simulink model "Project_Mobius"  (R2023b)
settings: Solver=ode4  StartTime=0.0  StopTime=100  FixedStep=5e-3  RelTol=1e-3
values from neighbouring files (symbols this model uses):
  aileron_stuck = 0.1    [fault_insertion.m]
  aircraft_b = 2    [initial.m]
  aircraft_c = 0.275    [initial.m]
  aircraft_mass = 6.031    [initial.m]
  c1 = ((Iyy - Izz)*Izz - Ixz*Ixz)/sigma    (= -0.404494382022)    [initial.m]
  c2 = ((Ixx - Iyy + Izz)*Ixz)/sigma    (= 0)    [initial.m]
  c3 = Izz/sigma    (= 3.74531835206)    [initial.m]
  c4 = Ixz/sigma    (= 0)    [initial.m]
  c5 = (Izz - Ixx)/Iyy    (= 0.404494382022)    [initial.m]
  c6 = Ixz/Iyy    (= 0)    [initial.m]
  c7 = 1/Iyy    (= 3.74531835206)    [initial.m]
  c8 = (Ixx*(Ixx - Iyy) + Ixz*Ixz)/sigma    (= 0)    [initial.m]
  c9 = Ixx/sigma    (= 2.66666666667)    [initial.m]
  CD_fuselage = 0.027    [initial.m]
  CdDa = 0.092132    [initial.m]
  CdDe = 0.016043    [initial.m]
  CdDr = 0.0097403    [initial.m]
  CDmin = 0.06047    [initial.m]
  CL0 = 0.81857    [initial.m]
  CL_CDmin = 0.4806    [initial.m]
  CLa = 4.09127    [initial.m]
  CLa_dot = 0    [initial.m]
  Clb = -0.00161    [initial.m]
  ClDa = 0.286593    [initial.m]
  CLDa = -0.85291    [initial.m]
  CLDe = 0.50787    [initial.m]
  ClDr = 0.013407    [initial.m]
  Clp = -0.47584    [initial.m]
  CLq = 7.31097    [initial.m]
  Clr = 0.27153    [initial.m]
  Cm0 = 0.00763    [initial.m]
  Cma = -1.76966    [initial.m]
  CmDe = -1.83747    [initial.m]
  Cmq = -19.22663    [initial.m]
  Cnb = 0.0918    [initial.m]
  CnDa = 0.0049274    [initial.m]
  CnDr = -0.067036    [initial.m]
  Cnp = -0.13267    [initial.m]
  Cnr = -0.08829    [initial.m]
  CYb = -0.00157    [initial.m]
  CYDr = 0.128915    [initial.m]
  CYp = -0.00157    [initial.m]
  CYr = 0.18368    [initial.m]
  elevator_stuck = 0    [fault_insertion.m]
  fault_time_start = 1    [fault_insertion.m]
  flight_mode = 1    [initial.m]
  g = 9.8060    (= 9.806)    [initial.m]
  init_alpha = alpha_trim    (= 0)    [initial.m]
  init_h = 10    [initial.m]
  init_p = 0    [initial.m]
  init_phi = 0    [initial.m]
  init_psi = 0    [initial.m]
  init_q = 0    [initial.m]
  init_r = 0    [initial.m]
  init_theta = init_alpha    (= 0)    [initial.m]
  init_u = Vb(1)    [initial.m]
  init_v = Vb(2)    [initial.m]
  init_w = Vb(3)    [initial.m]
  init_x = 0    [initial.m]
  init_y = 0    [initial.m]
  K = 0.1328    [initial.m]
  Max_RPM = 10000    [initial.m]
  p_sensor_fault = 0    [fault_insertion.m]
  phi_sensor_fault = 0    [fault_insertion.m]
  PropDiameter = 0.3052    [initial.m]
  psi_sensor_fault = 0    [fault_insertion.m]
  q_sensor_fault = 0    [fault_insertion.m]
  r_sensor_fault = 0    [fault_insertion.m]
  rho = 1.2250    (= 1.225)    [initial.m]
  rotor1_direction = 1    [initial.m]
  rotor1_fail = 0    [fault_insertion.m]
  rotor2_direction = -1    [initial.m]
  rotor2_fail = 0    [fault_insertion.m]
  rotor3_direction = -1    [initial.m]
  rotor3_fail = 0    [fault_insertion.m]
  rotor4_direction = 1    [initial.m]
  rotor4_fail = 0    [fault_insertion.m]
  rotor_arm1 = [0.375,0.375,0]    [initial.m]
  rotor_arm2 = [0.375,-0.375,0]    [initial.m]
  rotor_arm3 = [-0.375,-0.375,0]    [initial.m]
  rotor_arm4 = [-0.375,0.375,0]    [initial.m]
  RPM1_init = rotor_n * 60    (= 5940)    [initial.m]
  RPM2_init = rotor_n * 60    (= 5940)    [initial.m]
  RPM3_init = 0    [initial.m]
  RPM4_init = 0    [initial.m]
  rudder_stuck = 0    [fault_insertion.m]
  theta_sensor_fault = 0    [fault_insertion.m]
  tilt1_fail = 0    [fault_insertion.m]
  tilt1_init = lambda    [initial.m]
  tilt2_fail = 0    [fault_insertion.m]
  tilt2_init = lambda    [initial.m]
  tilt3_init = 0    [initial.m]
  tilt4_init = 0    [initial.m]
  u_sensor_fault = 0    [fault_insertion.m]
  v_sensor_fault = 0    [fault_insertion.m]
  w_sensor_fault = 0    [fault_insertion.m]
undefined symbols (not defined in the file or in its folder): FixedWingMission, HoverMission
libraries: slpidlib x20, simulink_extras x12, simulink x7, aerolibasang x6, matrix_library x4, uavalgslib x4, sharedutil x1, sharedtransform x1
(part 3 of 4)

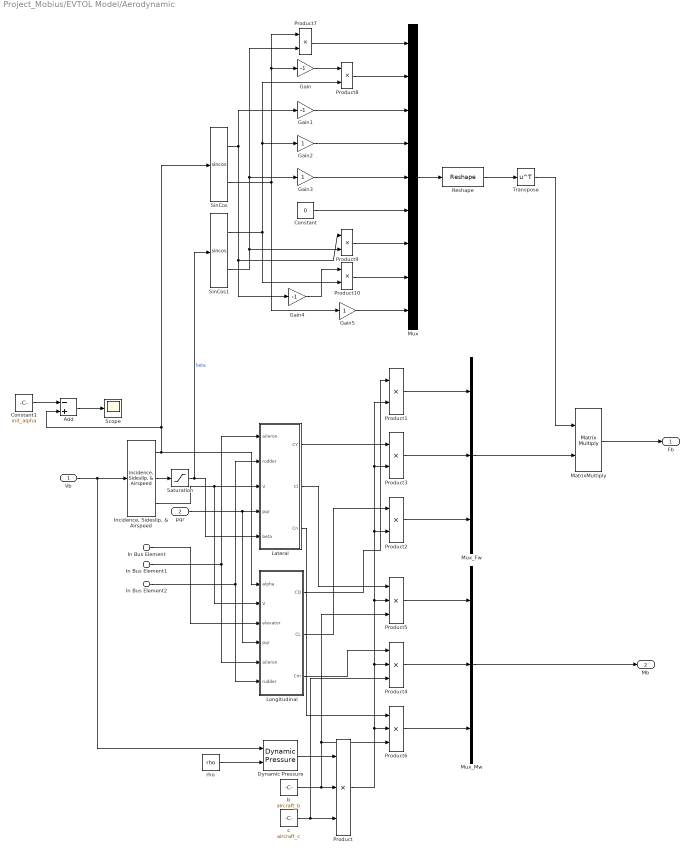
== system Project_Mobius/EVTOL Model/Aerodynamic ==
  Vb : Inport
  pqr : Inport  Port=2
  In Bus Element : Inport  Port=3  PortName=CtrlSurfaces  Element=Elevator
  In Bus Element1 : Inport  Port=3  PortName=CtrlSurfaces  Element=Aileron
  In Bus Element2 : Inport  Port=3  PortName=CtrlSurfaces  Element=Rudder
  Add : Sum  Inputs=-+
  Constant : Constant  Value=0
  Constant1 : Constant  Value=init_alpha
  Dynamic Pressure : aerolibasang/Dynamic Pressure
  Gain : Gain  Gain=-1
  Gain1 : Gain  Gain=-1
  Gain2 : Gain
  Gain3 : Gain
  Gain4 : Gain  Gain=-1
  Gain5 : Gain
  "Incidence, Sideslip, & Airspeed" : aerolibasang/Incidence, Sideslip, & Airspeed
  Lateral : Subsystem
  Longitudinal : Subsystem
  MatrixMultiply : Product  Multiplication=Matrix(*)
  Mux : Mux  Inputs=9
  Mux_Fw : Mux  Inputs=3
  Mux_Mw : Mux  Inputs=3
  Product{,4..6} (4 alike) : Product  Inputs=3
  Product{1..3,7..10} (7 alike) : Product
  Reshape : Reshape  OutputDimensionality=Customize  OutputDimensions=[3,3]
  Saturation : Saturate  UpperLimit=14*pi/180  LowerLimit=-14*pi/180
  Scope : Scope
  SinCos : Trigonometry  Operator=sincos
  SinCos1 : Trigonometry  Operator=sincos
  Transpose : Math  Operator=transpose
  b : Constant  Value=aircraft_b
  c : Constant  Value=aircraft_c
  rho : Constant  Value=rho
  Fb : Outport
  Mb : Outport  Port=2
  wires:
  Vb/1 -> "Incidence, Sideslip, & Airspeed"/1, Dynamic Pressure/1
  rho/1 -> Dynamic Pressure/2
  In Bus Element1/1 -> Longitudinal/5(aileron), Lateral/1(aileron)
  In Bus Element2/1 -> Longitudinal/6(rudder), Lateral/2(rudder)
  "Incidence, Sideslip, & Airspeed"/3 -> Longitudinal/2(V), Lateral/3(V)
  pqr/1 -> Longitudinal/4(pqr), Lateral/4(pqr)
  "Incidence, Sideslip, & Airspeed"/2 -> Saturation/1
  "Incidence, Sideslip, & Airspeed"/1 -> Add/2, SinCos/1, Longitudinal/1(alpha)
  In Bus Element/1 -> Longitudinal/3(elevator)
  Dynamic Pressure/1 -> Product/1
  b/1 -> Product6/3, Product5/3, Product/2
  c/1 -> Product4/3, Product/3
  Longitudinal/1(CD) -> Product1/1
  Product/1 -> Product2/2, Product3/2, Product1/2, Product5/2, Product4/2, Product6/2
  Longitudinal/2(CL) -> Product2/1
  Lateral/1(CY) -> Product3/1
  Longitudinal/3(Cm) -> Product4/1
  Lateral/2(Cl) -> Product5/1
  Lateral/3(Cn) -> Product6/1
  Product3/1 -> Mux_Fw/2
  Product2/1 -> Mux_Fw/3
  Product1/1 -> Mux_Fw/1
  Mux_Fw/1 -> MatrixMultiply/2
  Product5/1 -> Mux_Mw/1
  Product4/1 -> Mux_Mw/2
  Product6/1 -> Mux_Mw/3
  SinCos/2 -> Gain5/1, Gain/1, Product7/1
  SinCos1/2 -> Product9/2, Gain3/1, Product7/2
  Gain/1 -> Product8/1
  SinCos1/1 -> Product10/2, Gain2/1, Product8/2
  SinCos/1 -> Gain1/1, Product9/1, Gain4/1
  Gain4/1 -> Product10/1
  Product7/1 -> Mux/1
  Product8/1 -> Mux/2
  Gain1/1 -> Mux/3
  Gain2/1 -> Mux/4
  Gain3/1 -> Mux/5
  Constant/1 -> Mux/6
  Product9/1 -> Mux/7
  Product10/1 -> Mux/8
  Gain5/1 -> Mux/9
  Mux/1 -> Reshape/1
  MatrixMultiply/1 -> Fb/1
  Reshape/1 -> Transpose/1
  Transpose/1 -> MatrixMultiply/1
  Mux_Mw/1 -> Mb/1
  Saturation/1 -> SinCos1/1, Lateral/5(beta)  "beta"
  Constant1/1 -> Add/1
  Add/1 -> Scope/1

== system Project_Mobius/EVTOL Model/Fuselage Drag ==
  Vb : Inport
  Add : Sum  Inputs=+++
  Constant : Constant  Value=CD_fuselage
  Demux : Demux  Outputs=3
  Gain : Gain  Gain=-1
  Product : Product
  Product1 : Product
  Sqrt : Sqrt
  Square : Math  Operator=square
  Square1 : Math  Operator=square
  Square2 : Math  Operator=square
  FD,fuselage : Outport
  wires:
  Vb/1 -> Product1/2, Demux/1
  Demux/1 -> Square/1
  Demux/2 -> Square1/1
  Demux/3 -> Square2/1
  Square/1 -> Add/1
  Square1/1 -> Add/2
  Square2/1 -> Add/3
  Add/1 -> Sqrt/1
  Sqrt/1 -> Product/2
  Constant/1 -> Product/1
  Product/1 -> Product1/1
  Product1/1 -> Gain/1
  Gain/1 -> FD,fuselage/1

== system Project_Mobius/EVTOL Model/Gravity ==
  Attitude : Inport
  Demux : Demux  Outputs=3
  Gain : Gain  Gain=-1
  Gain1 : Gain  Gain=aircraft_mass*g
  Mux : Mux  Inputs=3
  Product : Product
  Product1 : Product
  SinCos : Trigonometry  Operator=sincos
  SinCos1 : Trigonometry  Operator=sincos
  Fb : Outport
  wires:
  Attitude/1 -> Demux/1
  Demux/1 -> SinCos/1
  Demux/2 -> SinCos1/1
  SinCos1/2 -> Product/2, Product1/1
  SinCos/1 -> Product/1
  SinCos/2 -> Product1/2
  SinCos1/1 -> Gain/1
  Gain/1 -> Mux/1
  Product/1 -> Mux/2
  Product1/1 -> Mux/3
  Mux/1 -> Gain1/1
  Gain1/1 -> Fb/1

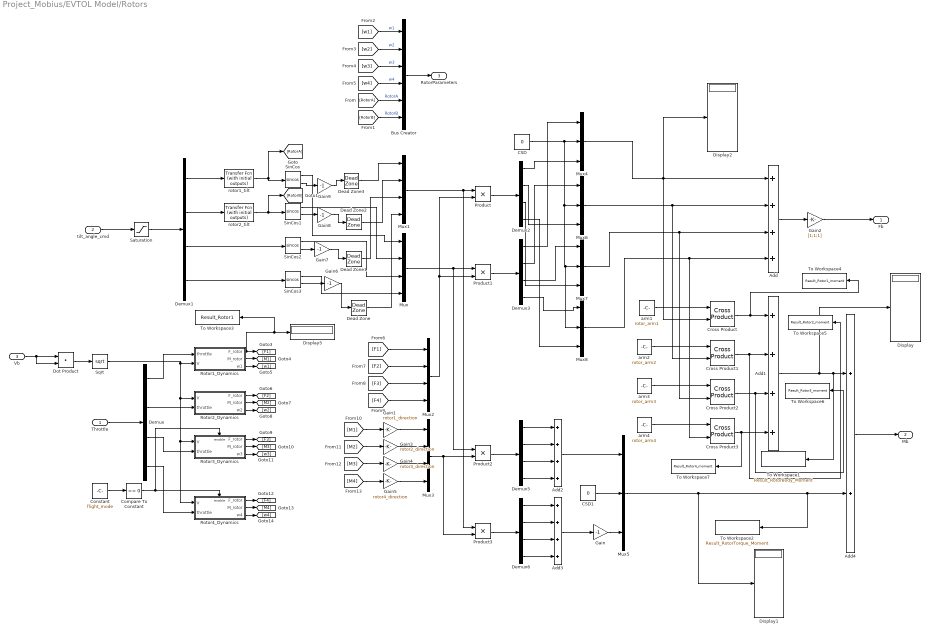
== system Project_Mobius/EVTOL Model/Rotors ==
  Throttle : Inport
  tilt_angle_cmd : Inport  Port=2
  Vb : Inport  Port=3
  Add{,1..3} (4 alike) : Sum  Inputs=++++
  Add4 : Sum
  Bus Creator : BusCreator  Inputs=6
  CSD : Constant  Value=0
  CSD1 : Constant  Value=0
  Compare To Constant : simulink/Logic and Bit Operations/Compare To Constant  relop===  const=0  OutDataTypeStr=boolean
  Constant : Constant  Value=flight_mode
  Cross Product{,1..3} (4 alike) : matrix_library/Cross Product
  Dead Zone{,1..3} (4 alike) : DeadZone  LowerValue=-cos(pi/2)  UpperValue=cos(pi/2)
  Demux{,1..3,5..6} (6 alike) : Demux
  Display{,1..2,5} (4 alike) : Display
  Dot Product : DotProduct  OutDataTypeStr=Inherit: Inherit via internal rule
  Gain{,6..9} (5 alike) : Gain  Gain=-1
  Gain1 : Gain  Gain=rotor1_direction
  Gain2 : Gain  Gain=[1;1;1]
  Gain3 : Gain  Gain=rotor2_direction
  Gain4 : Gain  Gain=rotor3_direction
  Gain5 : Gain  Gain=rotor4_direction
  Mux{,1..3} (4 alike) : Mux
  Mux{4..8} (5 alike) : Mux  Inputs=3
  Product{,1..3} (4 alike) : Product
  Rotor1_Dynamics : Subsystem
  Rotor2_Dynamics : Subsystem
  Rotor3_Dynamics : Subsystem
  Rotor4_Dynamics : Subsystem
  Saturation : Saturate  UpperLimit=90*pi/180  LowerLimit=-90*pi/180
  SinCos{,1..3} (4 alike) : Trigonometry  Operator=sincos
  Sqrt : Sqrt
  To Workspace1 : ToWorkspace  VariableName=Result_RotorBody_Moment  SampleTime=0.005
  To Workspace2 : ToWorkspace  VariableName=Result_RotorTorque_Moment  SampleTime=0.005
  To Workspace3 : ToWorkspace  VariableName=Result_Rotor1  SampleTime=0.005
  To Workspace4 : ToWorkspace  VariableName=Result_Rotor1_moment  SampleTime=0.005
  To Workspace5 : ToWorkspace  VariableName=Result_Rotor2_moment  SampleTime=0.005
  To Workspace6 : ToWorkspace  VariableName=Result_Rotor3_moment  SampleTime=0.005
  To Workspace7 : ToWorkspace  VariableName=Result_Rotor4_moment  SampleTime=0.005
  arm1 : Constant  Value=rotor_arm1
  arm2 : Constant  Value=rotor_arm2
  arm3 : Constant  Value=rotor_arm3
  arm4 : Constant  Value=rotor_arm4
  rotor1_tilt : simulink_extras/Additional Linear/Transfer Fcn (with initial outputs)  N=[1]  D="[0.1  1]"  Y0=tilt1_init  U0=tilt1_init
  rotor2_tilt : simulink_extras/Additional Linear/Transfer Fcn (with initial outputs)  N=[1]  D="[0.1  1]"  Y0=tilt2_init  U0=tilt2_init
  Fb : Outport
  Mb : Outport  Port=2
  RotorParameters : Outport  Port=3
  wires:
  Throttle/1 -> Demux/1
  Demux/1 -> Rotor1_Dynamics/1(throttle)
  Demux1/1 -> rotor1_tilt/1
  Demux1/2 -> rotor2_tilt/1
  tilt_angle_cmd/1 -> Saturation/1
  Saturation/1 -> Demux1/1
  rotor1_tilt/1 -> [RotorA], SinCos/1
  rotor2_tilt/1 -> [RotorB], SinCos1/1
  Demux1/3 -> SinCos2/1
  Demux1/4 -> SinCos3/1
  SinCos/1 -> Mux/1
  SinCos1/1 -> Mux/2
  SinCos2/1 -> Mux/3
  SinCos3/1 -> Mux/4
  SinCos1/2 -> Gain8/1
  SinCos3/2 -> Gain6/1
  Mux2/1 -> Product1/2, Product/2
  Product/1 -> Demux2/1
  Product1/1 -> Demux3/1
  Add/1 -> Gain2/1
  Mux3/1 -> Product3/2, Product2/2
  Mux/1 -> Product2/1, Product1/1
  Product2/1 -> Demux5/1
  Product3/1 -> Demux6/1
  Demux5/1 -> Add2/1
  Demux5/2 -> Add2/2
  Demux5/3 -> Add2/3
  Demux5/4 -> Add2/4
  Demux6/1 -> Add3/1
  Demux6/2 -> Add3/2
  Demux6/3 -> Add3/3
  Demux6/4 -> Add3/4
  Add3/1 -> Gain/1
  Add2/1 -> Mux5/1
  CSD1/1 -> Mux5/2
  CSD/1 -> Mux8/2, Mux7/2, Mux6/2, Mux4/2
  Mux7/1 -> Add/3, Cross Product2/2
  Mux8/1 -> Cross Product3/2, Add/4
  arm1/1 -> Cross Product/1
  arm2/1 -> Cross Product1/1
  Mux6/1 -> Add/2, Cross Product1/2
  arm3/1 -> Cross Product2/1
  arm4/1 -> Cross Product3/1
  Cross Product/1 -> To Workspace4/1, Add1/1
  Cross Product1/1 -> To Workspace5/1, Add1/2
  Cross Product2/1 -> To Workspace6/1, Add1/3
  Cross Product3/1 -> Add1/4, To Workspace7/1
  Add1/1 -> Display/1, To Workspace1/1, Add4/1
  Mux5/1 -> Display1/1, To Workspace2/1, Add4/2
  Add4/1 -> Mb/1
  Gain2/1 -> Fb/1
  Vb/1 -> Dot Product/2, Dot Product/1
  Dot Product/1 -> Sqrt/1
  Sqrt/1 -> Rotor4_Dynamics/1(V), Rotor3_Dynamics/1(V), Rotor2_Dynamics/1(V), Rotor1_Dynamics/2(V)
  Demux/2 -> Rotor2_Dynamics/2(throttle)
  Demux/3 -> Rotor3_Dynamics/2(throttle)
  Demux/4 -> Rotor4_Dynamics/2(throttle)
  Demux3/1 -> Mux4/1
  Demux3/2 -> Mux6/1
  Demux3/3 -> Mux7/1
  Demux3/4 -> Mux8/1
  Demux2/1 -> Mux4/3
  Demux2/2 -> Mux6/3
  Demux2/3 -> Mux7/3
  Demux2/4 -> Mux8/3
  Gain/1 -> Mux5/3
  Gain3/1 -> Mux3/2
  Gain4/1 -> Mux3/3
  Gain5/1 -> Mux3/4
  Mux1/1 -> Product3/1, Product/1
  Compare To Constant/1 -> Rotor4_Dynamics/Enable, Rotor3_Dynamics/Enable
  Dead Zone/1 -> Mux1/4
  SinCos2/2 -> Gain7/1
  Dead Zone1/1 -> Mux1/3
  Dead Zone2/1 -> Mux1/2
  Dead Zone3/1 -> Mux1/1
  [w1] -> Bus Creator/1  "w1"
  [w2] -> Bus Creator/2  "w2"
  [w3] -> Bus Creator/3  "w3"
  [w4] -> Bus Creator/4  "w4"
  [RotorA] -> Bus Creator/5  "RotorA"
  [RotorB] -> Bus Creator/6  "RotorB"
  Bus Creator/1 -> RotorParameters/1
  Gain1/1 -> Mux3/1
  Rotor1_Dynamics/1(F_rotor) -> To Workspace3/1, Display5/1, [F1]
  Rotor1_Dynamics/2(M_rotor) -> [M1]
  Rotor1_Dynamics/3(w1) -> [w1]
  Rotor2_Dynamics/1(F_rotor) -> [F2]
  Rotor2_Dynamics/2(M_rotor) -> [M2]
  Rotor2_Dynamics/3(w2) -> [w2]
  Rotor3_Dynamics/1(F_rotor) -> [F3]
  Rotor3_Dynamics/2(M_rotor) -> [M3]
  Rotor3_Dynamics/3(w3) -> [w3]
  Rotor4_Dynamics/1(F_rotor) -> [F4]
  Rotor4_Dynamics/2(M_rotor) -> [M4]
  Rotor4_Dynamics/3(w4) -> [w4]
  [F1] -> Mux2/1
  [F2] -> Mux2/2
  [F3] -> Mux2/3
  [F4] -> Mux2/4
  [M1] -> Gain1/1
  [M2] -> Gain3/1
  [M3] -> Gain4/1
  [M4] -> Gain5/1
  Gain6/1 -> Dead Zone/1
  Gain7/1 -> Dead Zone1/1
  Gain8/1 -> Dead Zone2/1
  SinCos/2 -> Gain9/1
  Gain9/1 -> Dead Zone3/1
  Mux4/1 -> Display2/1, Cross Product/2, Add/1
  Constant/1 -> Compare To Constant/1

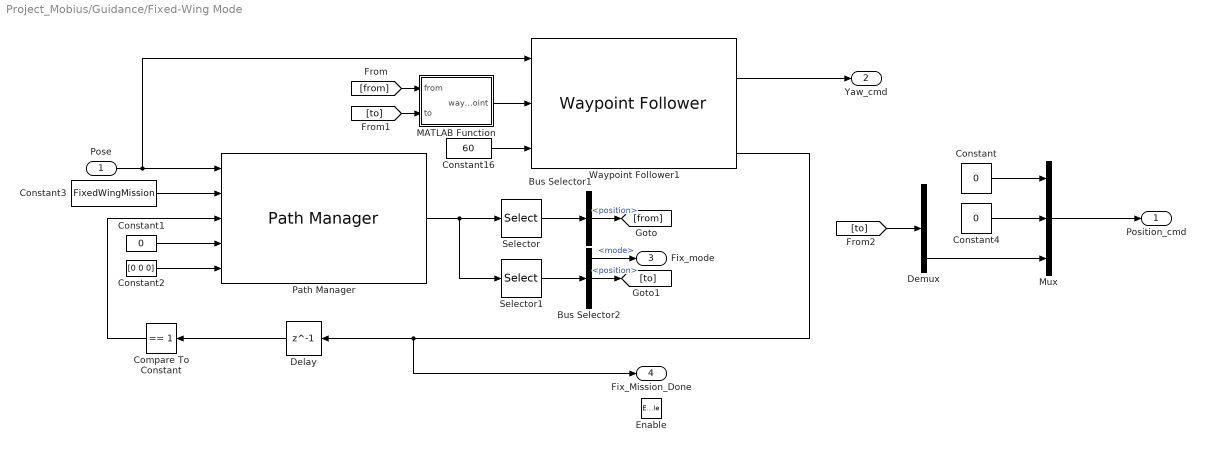
== system Project_Mobius/Guidance/Fixed-Wing Mode ==
  Pose : Inport
  Enable : EnablePort
  Bus Selector1 : BusSelector  OutputSignals=mode,position,params
  Bus Selector2 : BusSelector  OutputSignals=mode,position,params
  Compare To Constant : simulink/Logic and Bit Operations/Compare To Constant  relop===  const=1  OutDataTypeStr=boolean
  Constant : Constant  Value=0
  Constant1 : Constant  Value=0  OutDataTypeStr=uint8
  Constant16 : Constant  Value=60
  Constant2 : Constant  Value=[0 0 0]
  Constant3 : Constant  Value=FixedWingMission  OutDataTypeStr=Bus: doubleUAVPathManagerBus
  Constant4 : Constant  Value=0
  Delay : Delay  DelayLength=1  InitialCondition=0
  Demux : Demux  Outputs=3
  MATLAB Function : MATLAB Function  TreatAsAtomicUnit=on
  Mux : Mux  Inputs=3
  Path Manager : uavalgslib/Path Manager  UAVType=multirotor  LoiterRadius=25  dataType=double  inputBusName='doubleUAVPathManagerBus'  SimulateUsing=Interpreted execution
  Selector : Selector  InputPortWidth=2  IndexOptions=Index vector (dialog)  Indices=2  OutputSizes=1
  Selector1 : Selector  InputPortWidth=2  IndexOptions=Index vector (dialog)  Indices=1  OutputSizes=1
  Waypoint Follower1 : uavalgslib/Waypoint Follower  UAVType=fixed-wing  StartFrom=first  TransitionRadiusSource=internal  TransitionRadius=10  MinLookaheadDistance=60  YawInput=off  ShowCrossTrackErrorOutput=off  ShowStatusOutput=on  SimulateUsing=Code generation
  Position_cmd : Outport
  Yaw_cmd : Outport  Port=2
  Fix_mode : Outport  Port=3
  Fix_Mission_Done : Outport  Port=4
  wires:
  Pose/1 -> Waypoint Follower1/1, Path Manager/1
  MATLAB Function/1(waypoint) -> Waypoint Follower1/2
  Bus Selector1/2 -> [from]  "<position>"
  Waypoint Follower1/5 -> Fix_Mission_Done/1, Delay/1
  Delay/1 -> Compare To Constant/1
  Selector/1 -> Bus Selector1/1
  [from] -> MATLAB Function/1(from)
  Bus Selector2/2 -> [to]  "<position>"
  Constant1/1 -> Path Manager/4
  Constant3/1 -> Path Manager/2
  Constant16/1 -> Waypoint Follower1/3
  Path Manager/1 -> Selector1/1, Selector/1
  [to] -> MATLAB Function/2(to)
  Constant2/1 -> Path Manager/5
  Selector1/1 -> Bus Selector2/1
  Waypoint Follower1/2 -> Yaw_cmd/1
  Mux/1 -> Position_cmd/1
  Constant/1 -> Mux/1
  Constant4/1 -> Mux/2
  [to] -> Demux/1
  Demux/3 -> Mux/3
  Bus Selector2/1 -> Fix_mode/1  "<mode>"
  Compare To Constant/1 -> Path Manager/3

== system Project_Mobius/Guidance/Guidance Command ==
  Desired Position : Inport
  Desired_Course : Inport  Port=2
  Attitude Stablizer : Subsystem
  Bus Creator : BusCreator  Inputs=3
  Constant : Constant  Value=21
  Path_selector : Subsystem
  Command : Outport
  wires:
  Bus Creator/1 -> Command/1
  Attitude Stablizer/1(Attitude) -> [Attitude]  "Attitude"
  Path_selector/1(Xe_cmd) -> [Xe]  "Xe"
  [Attitude] -> Bus Creator/1  "Attitude"
  [Xe] -> Bus Creator/2  "Xe"
  Constant/1 -> Bus Creator/3  "Speed"
  Desired_Course/1 -> Path_selector/1(courseSP)
  Desired Position/1 -> Path_selector/2(positionSP)

== system Project_Mobius/Guidance/MultiRotor Mode ==
  Pose : Inport
  Enable : EnablePort
  Bus Selector1 : BusSelector  OutputSignals=mode,position,params
  Bus Selector2 : BusSelector  OutputSignals=mode,position,params
  Compare To Constant : simulink/Logic and Bit Operations/Compare To Constant  relop===  const=1  OutDataTypeStr=boolean
  Constant : Constant  Value=5
  Constant1 : Constant  Value=0  OutDataTypeStr=uint8
  Constant16 : Constant  Value=5
  Constant2 : Constant  Value=[0 0 0]
  Constant3 : Constant  Value=HoverMission  OutDataTypeStr=Bus: doubleUAVPathManagerBus
  Data Type Conversion : DataTypeConversion  OutDataTypeStr=uint8  SaturateOnIntegerOverflow=off  RndMeth=Floor
  Delay : Delay  DelayLength=1  InitialCondition=0
  Dist2WP : Subsystem
  MATLAB Function : MATLAB Function  TreatAsAtomicUnit=on
  Path Manager : uavalgslib/Path Manager  UAVType=multirotor  LoiterRadius=25  dataType=double  inputBusName='doubleUAVPathManagerBus'  SimulateUsing=Interpreted execution
  Relational Operator1 : RelationalOperator  OutDataTypeStr=boolean  RndMeth=Simplest  InputSameDT=off
  Selector : Selector  InputPortWidth=2  IndexOptions=Index vector (dialog)  Indices=2  OutputSizes=1
  Selector1 : Selector  InputPortWidth=2  IndexOptions=Index vector (dialog)  Indices=1  OutputSizes=1
  Waypoint Follower1 : uavalgslib/Waypoint Follower  UAVType=multirotor  StartFrom=closest  TransitionRadiusSource=internal  TransitionRadius=1  MinLookaheadDistance=0.1  YawInput=on  ShowCrossTrackErrorOutput=off  ShowStatusOutput=off  SimulateUsing=Code generation
  Position_cmd : Outport
  Yaw_cmd : Outport  Port=2
  Hover_mode : Outport  Port=3
  Hover_Mission_Done : Outport  Port=4
  wires:
  Pose/1 -> Dist2WP/3(Pose), Waypoint Follower1/1, Path Manager/1
  MATLAB Function/1(waypoint) -> Waypoint Follower1/2
  Relational Operator1/1 -> Data Type Conversion/1
  Bus Selector1/2 -> [from]  "<position>"
  Data Type Conversion/1 -> Hover_Mission_Done/1, Delay/1
  Compare To Constant/1 -> Path Manager/3
  Selector/1 -> Dist2WP/1(FromWP), Bus Selector1/1
  [from] -> MATLAB Function/1(from)
  Delay/1 -> Compare To Constant/1
  Bus Selector2/2 -> [to]  "<position>"
  Constant1/1 -> Path Manager/4
  Constant3/1 -> Path Manager/2
  Constant/1 -> Relational Operator1/1
  Dist2WP/1(Dist) -> Relational Operator1/2
  Constant16/1 -> Waypoint Follower1/3
  Path Manager/1 -> Selector1/1, Selector/1
  [to] -> MATLAB Function/2(to)
  Constant2/1 -> Path Manager/5
  Bus Selector2/1 -> Hover_mode/1  "<mode>"
  Selector1/1 -> Bus Selector2/1, Dist2WP/2(ToWP)
  Waypoint Follower1/1 -> Position_cmd/1
  Waypoint Follower1/3 -> Yaw_cmd/1

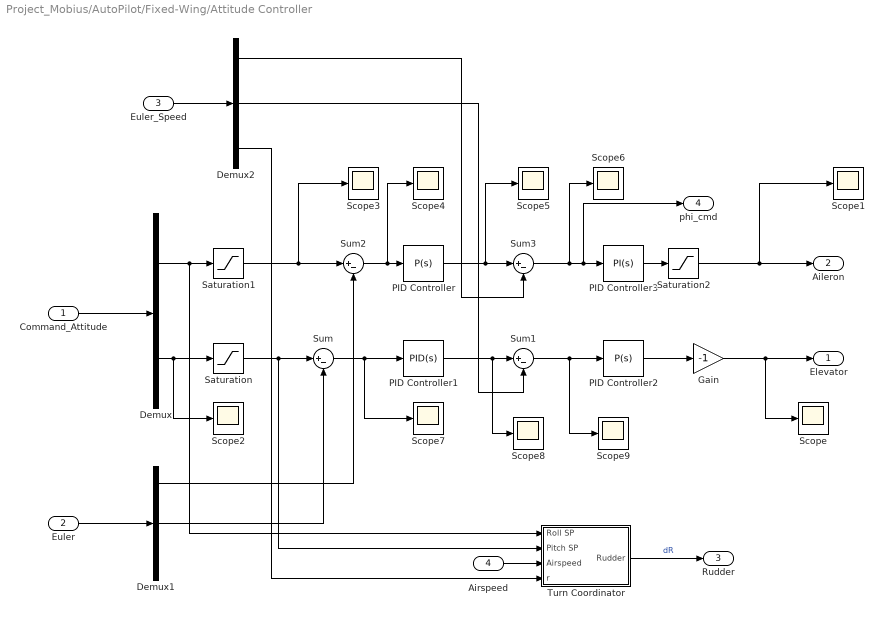
== system Project_Mobius/AutoPilot/Fixed-Wing/Attitude Controller ==
  Command_Attitude : Inport
  Euler : Inport  Port=2
  Euler_Speed : Inport  Port=3
  Airspeed : Inport  Port=4
  Demux : Demux  Outputs=2
  Demux1 : Demux  Outputs=3
  Demux2 : Demux  Outputs=3
  Gain : Gain  Gain=-1
  PID Controller : slpidlib/PID Controller  Controller=P  Form=Parallel  TimeDomain=Continuous-time  UseExternalTs=off  SampleTime=-1  IntegratorMethod=Forward Euler  FilterMethod=Forward Euler  ControllerParametersSource=internal  P=2  I=1  UseKiTs=off  D=0  N=100  UseFilter=on  TunerSelectOption=Transfer Function Based (PID Tuner App)  InitialConditionSource=internal  InitialConditionForIntegrator=0  InitialConditionForFilter=0  DifferentiatorICPrevScaledInput=0  ExternalReset=none  TrackingMode=off  Kt=1  LimitOutput=on  SatLimitsSource=internal  UpperSaturationLimit=1.2277  LowerSaturationLimit=-1.2277  LinearizeAsGain=on  AntiWindupMode=none  Kb=1  LimitIntegrator=off  UpperIntegratorSaturationLimit=inf  LowerIntegratorSaturationLimit=-inf  POutMin=[]  POutMax=[]  IOutMin=[]  IOutMax=[]  DOutMin=[]  DOutMax=[]  NOutMin=[]  NOutMax=[]  SumOutMin=[]  SumOutMax=[]  SaturationOutMin=[]  SaturationOutMax=[]  PParamMin=[]  PParamMax=[]  IParamMin=[]  IParamMax=[]  DParamMin=[]  DParamMax=[]  NParamMin=[]  NParamMax=[]  KbParamMin=[]  KbParamMax=[]  KtParamMin=[]  KtParamMax=[]  KbOutMin=[]  KbOutMax=[]  KtOutMin=[]  KtOutMax=[]  IntegratorOutMin=[]  IntegratorOutMax=[]  FilterOutMin=[]  FilterOutMax=[]  SumI1OutMin=[]  SumI1OutMax=[]  SumI2OutMin=[]  SumI2OutMax=[]  SumI3OutMin=[]  SumI3OutMax=[]  SumI4OutMin=[]  SumI4OutMax=[]  SumDOutMin=[]  SumDOutMax=[]  DifferentiatorOutMin=[]  DifferentiatorOutMax=[]  FilterDiffOutCoefMin=[]  FilterDiffOutCoefMax=[]  ReciprocalOutMin=[]  ReciprocalOutMax=[]  SumDenOutMin=[]  SumDenOutMax=[]  SumNumOutMin=[]  SumNumOutMax=[]  DivideOutMin=[]  DivideOutMax=[]  UdiffTsProdOutMin=[]  UdiffTsProdOutMax=[]  NTsProdOutMin=[]  NTsProdOutMax=[]  UintegralTsProdOutMin=[]  UintegralTsProdOutMax=[]  UngainTsProdOutMin=[]  UngainTsProdOutMax=[]  ClampingZeroOutDataTypeStr=Inherit: Inherit via back propagation  ClampingZeroOutMin=[]  ClampingZeroOutMax=[]  FilterDenConstantOutDataTypeStr=Inherit: Inherit via back propagation  FilterDenConstantOutMin=[]  FilterDenConstantOutMax=[]  PCopyOutDataTypeStr=Inherit: Inherit via back propagation  PCopyOutMin=[]  PCopyOutMax=[]  NCopyOutDataTypeStr=Inherit: Inherit via back propagation  NCopyOutMin=[]  NCopyOutMax=[]  IntegratorContinuousStateAttributes=''  IntegratorStateMustResolveToSignalObject=off  IntegratorRTWStateStorageClass=Auto  FilterContinuousStateAttributes=''  FilterStateMustResolveToSignalObject=off  FilterRTWStateStorageClass=Auto  ParallelPVariant=InternalParameters  IdealPVariant=Disabled  IVariant=Disabled  DVariant=Disabled  IntegratorVariant=Disabled  SatVariant=Enabled  AWVariant=Disabled  PCopyVariant=Disabled  TRVariant=Disabled  FdbkBlocksVariant=Forward  IdealPFdbkVariant=Disabled  SatFdbkVariant=Disabled  DerivativeFilterVariant=Disabled  NVariant=Disabled  NCopyVariant=Disabled_SignalSpec  FilterICVariant=Disabled  IntegratorICVariant=Disabled  ExternalResetVariant=Disabled  TRSumVariant=Passthrough  SumFdbkVariant=Disabled  SumVariant=Passthrough_P  TsampFilterVariant=InternalTs  TsampNgainVariant=Passthrough  TsampIntegralVariant=Disabled_SignalSpec  ExternalSaturationOutDataTypeStr=Inherit: Same as second input
  PID Controller1 : slpidlib/PID Controller  Controller=PID  Form=Parallel  TimeDomain=Continuous-time  UseExternalTs=off  SampleTime=0.05  IntegratorMethod=Forward Euler  FilterMethod=Forward Euler  ControllerParametersSource=internal  P=10  I=0.1  UseKiTs=off  D=0  N=2.2  UseFilter=on  TunerSelectOption=Transfer Function Based (PID Tuner App)  InitialConditionSource=internal  InitialConditionForIntegrator=0  InitialConditionForFilter=0  DifferentiatorICPrevScaledInput=0  ExternalReset=none  TrackingMode=off  Kt=1  LimitOutput=on  SatLimitsSource=internal  UpperSaturationLimit=inf  LowerSaturationLimit=-inf  LinearizeAsGain=on  AntiWindupMode=clamping  Kb=1  LimitIntegrator=off  UpperIntegratorSaturationLimit=inf  LowerIntegratorSaturationLimit=-inf  POutMin=[]  POutMax=[]  IOutMin=[]  IOutMax=[]  DOutMin=[]  DOutMax=[]  NOutMin=[]  NOutMax=[]  SumOutMin=[]  SumOutMax=[]  SaturationOutMin=[]  SaturationOutMax=[]  PParamMin=[]  PParamMax=[]  IParamMin=[]  IParamMax=[]  DParamMin=[]  DParamMax=[]  NParamMin=[]  NParamMax=[]  KbParamMin=[]  KbParamMax=[]  KtParamMin=[]  KtParamMax=[]  KbOutMin=[]  KbOutMax=[]  KtOutMin=[]  KtOutMax=[]  IntegratorOutMin=[]  IntegratorOutMax=[]  FilterOutMin=[]  FilterOutMax=[]  SumI1OutMin=[]  SumI1OutMax=[]  SumI2OutMin=[]  SumI2OutMax=[]  SumI3OutMin=[]  SumI3OutMax=[]  SumI4OutMin=[]  SumI4OutMax=[]  SumDOutMin=[]  SumDOutMax=[]  DifferentiatorOutMin=[]  DifferentiatorOutMax=[]  FilterDiffOutCoefMin=[]  FilterDiffOutCoefMax=[]  ReciprocalOutMin=[]  ReciprocalOutMax=[]  SumDenOutMin=[]  SumDenOutMax=[]  SumNumOutMin=[]  SumNumOutMax=[]  DivideOutMin=[]  DivideOutMax=[]  UdiffTsProdOutMin=[]  UdiffTsProdOutMax=[]  NTsProdOutMin=[]  NTsProdOutMax=[]  UintegralTsProdOutMin=[]  UintegralTsProdOutMax=[]  UngainTsProdOutMin=[]  UngainTsProdOutMax=[]  ClampingZeroOutDataTypeStr=Inherit: Inherit via back propagation  ClampingZeroOutMin=[]  ClampingZeroOutMax=[]  FilterDenConstantOutDataTypeStr=Inherit: Inherit via back propagation  FilterDenConstantOutMin=[]  FilterDenConstantOutMax=[]  PCopyOutDataTypeStr=Inherit: Inherit via back propagation  PCopyOutMin=[]  PCopyOutMax=[]  NCopyOutDataTypeStr=Inherit: Inherit via back propagation  NCopyOutMin=[]  NCopyOutMax=[]  IntegratorContinuousStateAttributes=''  IntegratorStateMustResolveToSignalObject=off  IntegratorRTWStateStorageClass=Auto  FilterContinuousStateAttributes=''  FilterStateMustResolveToSignalObject=off  FilterRTWStateStorageClass=Auto  ParallelPVariant=InternalParameters  IdealPVariant=Disabled  IVariant=InternalParameters  DVariant=InternalParameters  IntegratorVariant=Continuous  SatVariant=Enabled  AWVariant=ContClampingParallel  PCopyVariant=Disabled  TRVariant=Disabled  FdbkBlocksVariant=Forward  IdealPFdbkVariant=Disabled  SatFdbkVariant=Disabled  DerivativeFilterVariant=ContFilter  NVariant=InternalParameters  NCopyVariant=Disabled  FilterICVariant=InternalICsFilter  IntegratorICVariant=InternalICs  ExternalResetVariant=Disabled  TRSumVariant=Passthrough  SumFdbkVariant=Disabled  SumVariant=Sum_PID  TsampFilterVariant=InternalTs  TsampNgainVariant=Passthrough  TsampIntegralVariant=Disabled_SignalSpec  ExternalSaturationOutDataTypeStr=Inherit: Same as second input
  PID Controller2 : slpidlib/PID Controller  Controller=P  Form=Parallel  TimeDomain=Continuous-time  UseExternalTs=off  SampleTime=0.05  IntegratorMethod=Forward Euler  FilterMethod=Forward Euler  ControllerParametersSource=internal  P=0.15  I=0  UseKiTs=off  D=0  N=2  UseFilter=on  TunerSelectOption=Transfer Function Based (PID Tuner App)  InitialConditionSource=internal  InitialConditionForIntegrator=0  InitialConditionForFilter=0  DifferentiatorICPrevScaledInput=0  ExternalReset=none  TrackingMode=off  Kt=1  LimitOutput=on  SatLimitsSource=internal  UpperSaturationLimit=inf  LowerSaturationLimit=-inf  LinearizeAsGain=on  AntiWindupMode=none  Kb=1  LimitIntegrator=off  UpperIntegratorSaturationLimit=inf  LowerIntegratorSaturationLimit=-inf  POutMin=[]  POutMax=[]  IOutMin=[]  IOutMax=[]  DOutMin=[]  DOutMax=[]  NOutMin=[]  NOutMax=[]  SumOutMin=[]  SumOutMax=[]  SaturationOutMin=[]  SaturationOutMax=[]  PParamMin=[]  PParamMax=[]  IParamMin=[]  IParamMax=[]  DParamMin=[]  DParamMax=[]  NParamMin=[]  NParamMax=[]  KbParamMin=[]  KbParamMax=[]  KtParamMin=[]  KtParamMax=[]  KbOutMin=[]  KbOutMax=[]  KtOutMin=[]  KtOutMax=[]  IntegratorOutMin=[]  IntegratorOutMax=[]  FilterOutMin=[]  FilterOutMax=[]  SumI1OutMin=[]  SumI1OutMax=[]  SumI2OutMin=[]  SumI2OutMax=[]  SumI3OutMin=[]  SumI3OutMax=[]  SumI4OutMin=[]  SumI4OutMax=[]  SumDOutMin=[]  SumDOutMax=[]  DifferentiatorOutMin=[]  DifferentiatorOutMax=[]  FilterDiffOutCoefMin=[]  FilterDiffOutCoefMax=[]  ReciprocalOutMin=[]  ReciprocalOutMax=[]  SumDenOutMin=[]  SumDenOutMax=[]  SumNumOutMin=[]  SumNumOutMax=[]  DivideOutMin=[]  DivideOutMax=[]  UdiffTsProdOutMin=[]  UdiffTsProdOutMax=[]  NTsProdOutMin=[]  NTsProdOutMax=[]  UintegralTsProdOutMin=[]  UintegralTsProdOutMax=[]  UngainTsProdOutMin=[]  UngainTsProdOutMax=[]  ClampingZeroOutDataTypeStr=Inherit: Inherit via back propagation  ClampingZeroOutMin=[]  ClampingZeroOutMax=[]  FilterDenConstantOutDataTypeStr=Inherit: Inherit via back propagation  FilterDenConstantOutMin=[]  FilterDenConstantOutMax=[]  PCopyOutDataTypeStr=Inherit: Inherit via back propagation  PCopyOutMin=[]  PCopyOutMax=[]  NCopyOutDataTypeStr=Inherit: Inherit via back propagation  NCopyOutMin=[]  NCopyOutMax=[]  IntegratorContinuousStateAttributes=''  IntegratorStateMustResolveToSignalObject=off  IntegratorRTWStateStorageClass=Auto  FilterContinuousStateAttributes=''  FilterStateMustResolveToSignalObject=off  FilterRTWStateStorageClass=Auto  ParallelPVariant=InternalParameters  IdealPVariant=Disabled  IVariant=Disabled  DVariant=Disabled  IntegratorVariant=Disabled  SatVariant=Enabled  AWVariant=Disabled  PCopyVariant=Disabled  TRVariant=Disabled  FdbkBlocksVariant=Forward  IdealPFdbkVariant=Disabled  SatFdbkVariant=Disabled  DerivativeFilterVariant=Disabled  NVariant=Disabled  NCopyVariant=Disabled_SignalSpec  FilterICVariant=Disabled  IntegratorICVariant=Disabled  ExternalResetVariant=Disabled  TRSumVariant=Passthrough  SumFdbkVariant=Disabled  SumVariant=Passthrough_P  TsampFilterVariant=InternalTs  TsampNgainVariant=Passthrough  TsampIntegralVariant=Disabled_SignalSpec  ExternalSaturationOutDataTypeStr=Inherit: Same as second input
  PID Controller3 : slpidlib/PID Controller  Controller=PI  Form=Parallel  TimeDomain=Continuous-time  UseExternalTs=off  SampleTime=-1  IntegratorMethod=Forward Euler  FilterMethod=Forward Euler  ControllerParametersSource=internal  P=0.4  I=0.8  UseKiTs=off  D=0  N=100  UseFilter=on  TunerSelectOption=Transfer Function Based (PID Tuner App)  InitialConditionSource=internal  InitialConditionForIntegrator=0  InitialConditionForFilter=0  DifferentiatorICPrevScaledInput=0  ExternalReset=none  TrackingMode=off  Kt=1  LimitOutput=on  SatLimitsSource=internal  UpperSaturationLimit=1  LowerSaturationLimit=-1  LinearizeAsGain=on  AntiWindupMode=clamping  Kb=1  LimitIntegrator=off  UpperIntegratorSaturationLimit=inf  LowerIntegratorSaturationLimit=-inf  POutMin=[]  POutMax=[]  IOutMin=[]  IOutMax=[]  DOutMin=[]  DOutMax=[]  NOutMin=[]  NOutMax=[]  SumOutMin=[]  SumOutMax=[]  SaturationOutMin=[]  SaturationOutMax=[]  PParamMin=[]  PParamMax=[]  IParamMin=[]  IParamMax=[]  DParamMin=[]  DParamMax=[]  NParamMin=[]  NParamMax=[]  KbParamMin=[]  KbParamMax=[]  KtParamMin=[]  KtParamMax=[]  KbOutMin=[]  KbOutMax=[]  KtOutMin=[]  KtOutMax=[]  IntegratorOutMin=[]  IntegratorOutMax=[]  FilterOutMin=[]  FilterOutMax=[]  SumI1OutMin=[]  SumI1OutMax=[]  SumI2OutMin=[]  SumI2OutMax=[]  SumI3OutMin=[]  SumI3OutMax=[]  SumI4OutMin=[]  SumI4OutMax=[]  SumDOutMin=[]  SumDOutMax=[]  DifferentiatorOutMin=[]  DifferentiatorOutMax=[]  FilterDiffOutCoefMin=[]  FilterDiffOutCoefMax=[]  ReciprocalOutMin=[]  ReciprocalOutMax=[]  SumDenOutMin=[]  SumDenOutMax=[]  SumNumOutMin=[]  SumNumOutMax=[]  DivideOutMin=[]  DivideOutMax=[]  UdiffTsProdOutMin=[]  UdiffTsProdOutMax=[]  NTsProdOutMin=[]  NTsProdOutMax=[]  UintegralTsProdOutMin=[]  UintegralTsProdOutMax=[]  UngainTsProdOutMin=[]  UngainTsProdOutMax=[]  ClampingZeroOutDataTypeStr=Inherit: Inherit via back propagation  ClampingZeroOutMin=[]  ClampingZeroOutMax=[]  FilterDenConstantOutDataTypeStr=Inherit: Inherit via back propagation  FilterDenConstantOutMin=[]  FilterDenConstantOutMax=[]  PCopyOutDataTypeStr=Inherit: Inherit via back propagation  PCopyOutMin=[]  PCopyOutMax=[]  NCopyOutDataTypeStr=Inherit: Inherit via back propagation  NCopyOutMin=[]  NCopyOutMax=[]  IntegratorContinuousStateAttributes=''  IntegratorStateMustResolveToSignalObject=off  IntegratorRTWStateStorageClass=Auto  FilterContinuousStateAttributes=''  FilterStateMustResolveToSignalObject=off  FilterRTWStateStorageClass=Auto  ParallelPVariant=InternalParameters  IdealPVariant=Disabled  IVariant=InternalParameters  DVariant=Disabled  IntegratorVariant=Continuous  SatVariant=Enabled  AWVariant=ContClampingParallel  PCopyVariant=Disabled  TRVariant=Disabled  FdbkBlocksVariant=Forward  IdealPFdbkVariant=Disabled  SatFdbkVariant=Disabled  DerivativeFilterVariant=Disabled  NVariant=Disabled  NCopyVariant=Disabled_SignalSpec  FilterICVariant=Disabled  IntegratorICVariant=InternalICs  ExternalResetVariant=Disabled  TRSumVariant=Passthrough  SumFdbkVariant=Disabled  SumVariant=Sum_PI  TsampFilterVariant=InternalTs  TsampNgainVariant=Passthrough  TsampIntegralVariant=Disabled_SignalSpec  ExternalSaturationOutDataTypeStr=Inherit: Same as second input
  Saturation : Saturate  UpperLimit=0.18  LowerLimit=-0.18
  Saturation1 : Saturate  UpperLimit=0.7  LowerLimit=-0.7
  Saturation2 : Saturate  UpperLimit=0.3  LowerLimit=-0.3
  Scope{,1..9} (10 alike) : Scope
  Sum{,1..3} (4 alike) : Sum  Inputs=|+-
  Turn Coordinator : Subsystem
  Elevator : Outport
  Aileron : Outport  Port=2
  Rudder : Outport  Port=3
  phi_cmd : Outport  Port=4
  wires:
  Command_Attitude/1 -> Demux/1
  Euler/1 -> Demux1/1
  Euler_Speed/1 -> Demux2/1
  Demux1/2 -> Sum/2
  Sum/1 -> Scope7/1, PID Controller1/1
  Demux/2 -> Scope2/1, Saturation/1
  PID Controller1/1 -> Scope8/1, Sum1/1
  Demux2/2 -> Sum1/2
  Sum1/1 -> Scope9/1, PID Controller2/1
  PID Controller2/1 -> Gain/1
  Gain/1 -> Scope/1, Elevator/1
  Demux1/1 -> Sum2/2
  Demux/1 -> Turn Coordinator/1(Roll SP), Saturation1/1
  Sum2/1 -> Scope4/1, PID Controller/1
  PID Controller/1 -> Scope5/1, Sum3/1
  Sum3/1 -> Scope6/1, phi_cmd/1, PID Controller3/1
  PID Controller3/1 -> Saturation2/1
  Demux2/1 -> Sum3/2
  Demux2/3 -> Turn Coordinator/4(r)
  Airspeed/1 -> Turn Coordinator/3(Airspeed)
  Turn Coordinator/1(Rudder) -> Rudder/1  "dR"
  Saturation/1 -> Turn Coordinator/2(Pitch SP), Sum/1
  Saturation1/1 -> Scope3/1, Sum2/1
  Saturation2/1 -> Scope1/1, Aileron/1

== system Project_Mobius/AutoPilot/Fixed-Wing/Position Controller ==
  Command_Xe : Inport
  Xe : Inport  Port=2
  Ve : Inport  Port=3
  GndSpeed : Inport  Port=4
  Course : Inport  Port=5
  Constant : Constant  Value=60
  Demux : Demux
  Demux1 : Demux  Outputs=3
  Demux2 : Demux  Outputs=3
  MATLAB Function : MATLAB Function  TreatAsAtomicUnit=on
  Mux : Mux  Inputs=2
  PID Controller : slpidlib/PID Controller  Controller=P  Form=Parallel  TimeDomain=Continuous-time  UseExternalTs=off  SampleTime=-1  IntegratorMethod=Forward Euler  FilterMethod=Forward Euler  ControllerParametersSource=internal  P=0.4  I=0.001  UseKiTs=off  D=0  N=100  UseFilter=on  TunerSelectOption=Transfer Function Based (PID Tuner App)  InitialConditionSource=internal  InitialConditionForIntegrator=0  InitialConditionForFilter=0  DifferentiatorICPrevScaledInput=0  ExternalReset=none  TrackingMode=off  Kt=1  LimitOutput=on  SatLimitsSource=internal  UpperSaturationLimit=3  LowerSaturationLimit=-3  LinearizeAsGain=on  AntiWindupMode=none  Kb=1  LimitIntegrator=off  UpperIntegratorSaturationLimit=inf  LowerIntegratorSaturationLimit=-inf  POutMin=[]  POutMax=[]  IOutMin=[]  IOutMax=[]  DOutMin=[]  DOutMax=[]  NOutMin=[]  NOutMax=[]  SumOutMin=[]  SumOutMax=[]  SaturationOutMin=[]  SaturationOutMax=[]  PParamMin=[]  PParamMax=[]  IParamMin=[]  IParamMax=[]  DParamMin=[]  DParamMax=[]  NParamMin=[]  NParamMax=[]  KbParamMin=[]  KbParamMax=[]  KtParamMin=[]  KtParamMax=[]  KbOutMin=[]  KbOutMax=[]  KtOutMin=[]  KtOutMax=[]  IntegratorOutMin=[]  IntegratorOutMax=[]  FilterOutMin=[]  FilterOutMax=[]  SumI1OutMin=[]  SumI1OutMax=[]  SumI2OutMin=[]  SumI2OutMax=[]  SumI3OutMin=[]  SumI3OutMax=[]  SumI4OutMin=[]  SumI4OutMax=[]  SumDOutMin=[]  SumDOutMax=[]  DifferentiatorOutMin=[]  DifferentiatorOutMax=[]  FilterDiffOutCoefMin=[]  FilterDiffOutCoefMax=[]  ReciprocalOutMin=[]  ReciprocalOutMax=[]  SumDenOutMin=[]  SumDenOutMax=[]  SumNumOutMin=[]  SumNumOutMax=[]  DivideOutMin=[]  DivideOutMax=[]  UdiffTsProdOutMin=[]  UdiffTsProdOutMax=[]  NTsProdOutMin=[]  NTsProdOutMax=[]  UintegralTsProdOutMin=[]  UintegralTsProdOutMax=[]  UngainTsProdOutMin=[]  UngainTsProdOutMax=[]  ClampingZeroOutDataTypeStr=Inherit: Inherit via back propagation  ClampingZeroOutMin=[]  ClampingZeroOutMax=[]  FilterDenConstantOutDataTypeStr=Inherit: Inherit via back propagation  FilterDenConstantOutMin=[]  FilterDenConstantOutMax=[]  PCopyOutDataTypeStr=Inherit: Inherit via back propagation  PCopyOutMin=[]  PCopyOutMax=[]  NCopyOutDataTypeStr=Inherit: Inherit via back propagation  NCopyOutMin=[]  NCopyOutMax=[]  IntegratorContinuousStateAttributes=''  IntegratorStateMustResolveToSignalObject=off  IntegratorRTWStateStorageClass=Auto  FilterContinuousStateAttributes=''  FilterStateMustResolveToSignalObject=off  FilterRTWStateStorageClass=Auto  ParallelPVariant=InternalParameters  IdealPVariant=Disabled  IVariant=Disabled  DVariant=Disabled  IntegratorVariant=Disabled  SatVariant=Enabled  AWVariant=Disabled  PCopyVariant=Disabled  TRVariant=Disabled  FdbkBlocksVariant=Forward  IdealPFdbkVariant=Disabled  SatFdbkVariant=Disabled  DerivativeFilterVariant=Disabled  NVariant=Disabled  NCopyVariant=Disabled_SignalSpec  FilterICVariant=Disabled  IntegratorICVariant=Disabled  ExternalResetVariant=Disabled  TRSumVariant=Passthrough  SumFdbkVariant=Disabled  SumVariant=Passthrough_P  TsampFilterVariant=InternalTs  TsampNgainVariant=Passthrough  TsampIntegralVariant=Disabled_SignalSpec  ExternalSaturationOutDataTypeStr=Inherit: Same as second input
  PID Controller1 : slpidlib/PID Controller  Controller=P  Form=Parallel  TimeDomain=Continuous-time  UseExternalTs=off  SampleTime=-1  IntegratorMethod=Forward Euler  FilterMethod=Forward Euler  ControllerParametersSource=internal  P=0.1  I=0.237648506119343  UseKiTs=off  D=0  N=100  UseFilter=on  TunerSelectOption=Transfer Function Based (PID Tuner App)  InitialConditionSource=internal  InitialConditionForIntegrator=0  InitialConditionForFilter=0  DifferentiatorICPrevScaledInput=0  ExternalReset=none  TrackingMode=off  Kt=1  LimitOutput=on  SatLimitsSource=internal  UpperSaturationLimit=0.1743  LowerSaturationLimit=-0.1743  LinearizeAsGain=on  AntiWindupMode=none  Kb=1  LimitIntegrator=off  UpperIntegratorSaturationLimit=inf  LowerIntegratorSaturationLimit=-inf  POutMin=[]  POutMax=[]  IOutMin=[]  IOutMax=[]  DOutMin=[]  DOutMax=[]  NOutMin=[]  NOutMax=[]  SumOutMin=[]  SumOutMax=[]  SaturationOutMin=[]  SaturationOutMax=[]  PParamMin=[]  PParamMax=[]  IParamMin=[]  IParamMax=[]  DParamMin=[]  DParamMax=[]  NParamMin=[]  NParamMax=[]  KbParamMin=[]  KbParamMax=[]  KtParamMin=[]  KtParamMax=[]  KbOutMin=[]  KbOutMax=[]  KtOutMin=[]  KtOutMax=[]  IntegratorOutMin=[]  IntegratorOutMax=[]  FilterOutMin=[]  FilterOutMax=[]  SumI1OutMin=[]  SumI1OutMax=[]  SumI2OutMin=[]  SumI2OutMax=[]  SumI3OutMin=[]  SumI3OutMax=[]  SumI4OutMin=[]  SumI4OutMax=[]  SumDOutMin=[]  SumDOutMax=[]  DifferentiatorOutMin=[]  DifferentiatorOutMax=[]  FilterDiffOutCoefMin=[]  FilterDiffOutCoefMax=[]  ReciprocalOutMin=[]  ReciprocalOutMax=[]  SumDenOutMin=[]  SumDenOutMax=[]  SumNumOutMin=[]  SumNumOutMax=[]  DivideOutMin=[]  DivideOutMax=[]  UdiffTsProdOutMin=[]  UdiffTsProdOutMax=[]  NTsProdOutMin=[]  NTsProdOutMax=[]  UintegralTsProdOutMin=[]  UintegralTsProdOutMax=[]  UngainTsProdOutMin=[]  UngainTsProdOutMax=[]  ClampingZeroOutDataTypeStr=Inherit: Inherit via back propagation  ClampingZeroOutMin=[]  ClampingZeroOutMax=[]  FilterDenConstantOutDataTypeStr=Inherit: Inherit via back propagation  FilterDenConstantOutMin=[]  FilterDenConstantOutMax=[]  PCopyOutDataTypeStr=Inherit: Inherit via back propagation  PCopyOutMin=[]  PCopyOutMax=[]  NCopyOutDataTypeStr=Inherit: Inherit via back propagation  NCopyOutMin=[]  NCopyOutMax=[]  IntegratorContinuousStateAttributes=''  IntegratorStateMustResolveToSignalObject=off  IntegratorRTWStateStorageClass=Auto  FilterContinuousStateAttributes=''  FilterStateMustResolveToSignalObject=off  FilterRTWStateStorageClass=Auto  ParallelPVariant=InternalParameters  IdealPVariant=Disabled  IVariant=Disabled  DVariant=Disabled  IntegratorVariant=Disabled  SatVariant=Enabled  AWVariant=Disabled  PCopyVariant=Disabled  TRVariant=Disabled  FdbkBlocksVariant=Forward  IdealPFdbkVariant=Disabled  SatFdbkVariant=Disabled  DerivativeFilterVariant=Disabled  NVariant=Disabled  NCopyVariant=Disabled_SignalSpec  FilterICVariant=Disabled  IntegratorICVariant=Disabled  ExternalResetVariant=Disabled  TRSumVariant=Passthrough  SumFdbkVariant=Disabled  SumVariant=Passthrough_P  TsampFilterVariant=InternalTs  TsampNgainVariant=Passthrough  TsampIntegralVariant=Disabled_SignalSpec  ExternalSaturationOutDataTypeStr=Inherit: Same as second input
  Scope{,1..4} (5 alike) : Scope
  Sum : Sum  Inputs=|+-
  Sum1 : Sum  Inputs=|+-
  Terminator : Terminator
  Unary Minus : UnaryMinus
  Attitude_command : Outport
  wires:
  Command_Xe/1 -> Demux/1
  Xe/1 -> Demux1/1
  Demux/3 -> Sum/1
  Demux1/3 -> Sum/2
  Sum/1 -> Scope/1, PID Controller/1
  PID Controller/1 -> Scope3/1, Sum1/1
  Ve/1 -> Demux2/1
  Demux2/3 -> Sum1/2
  Sum1/1 -> Scope2/1, PID Controller1/1
  MATLAB Function/2(rollSP) -> Scope1/1, Mux/1
  Mux/1 -> Attitude_command/1
  Unary Minus/1 -> Scope4/1, Mux/2
  GndSpeed/1 -> MATLAB Function/3(groundSpeed)
  Course/1 -> MATLAB Function/2(course)
  MATLAB Function/1(lacc) -> Terminator/1
  Constant/1 -> MATLAB Function/4(L1)
  Demux/4 -> MATLAB Function/1(courseSP)
  PID Controller1/1 -> Unary Minus/1

== system Project_Mobius/AutoPilot/Fixed-Wing/Speed Controller ==
  Command_Speed : Inport
  Vb : Inport  Port=2
  Add : Sum
  Constant : Constant  Value=RPM1_init/10000
  Constant1 : Constant  Value=0
  Constant2 : Constant  Value=0
  "Incidence, Sideslip, & Airspeed" : aerolibasang/Incidence, Sideslip, & Airspeed
  Mux : Mux
  PID Controller : slpidlib/PID Controller  Controller=P  Form=Parallel  TimeDomain=Continuous-time  UseExternalTs=off  SampleTime=-1  IntegratorMethod=Forward Euler  FilterMethod=Forward Euler  ControllerParametersSource=internal  P=10  I=6.43017159164334  UseKiTs=off  D=0.302363595518722  N=492.520175767548  UseFilter=on  TunerSelectOption=Transfer Function Based (PID Tuner App)  InitialConditionSource=internal  InitialConditionForIntegrator=0  InitialConditionForFilter=0  DifferentiatorICPrevScaledInput=0  ExternalReset=none  TrackingMode=off  Kt=1  LimitOutput=off  SatLimitsSource=internal  UpperSaturationLimit=inf  LowerSaturationLimit=-inf  LinearizeAsGain=on  AntiWindupMode=none  Kb=1  LimitIntegrator=off  UpperIntegratorSaturationLimit=inf  LowerIntegratorSaturationLimit=-inf  POutMin=[]  POutMax=[]  IOutMin=[]  IOutMax=[]  DOutMin=[]  DOutMax=[]  NOutMin=[]  NOutMax=[]  SumOutMin=[]  SumOutMax=[]  SaturationOutMin=[]  SaturationOutMax=[]  PParamMin=[]  PParamMax=[]  IParamMin=[]  IParamMax=[]  DParamMin=[]  DParamMax=[]  NParamMin=[]  NParamMax=[]  KbParamMin=[]  KbParamMax=[]  KtParamMin=[]  KtParamMax=[]  KbOutMin=[]  KbOutMax=[]  KtOutMin=[]  KtOutMax=[]  IntegratorOutMin=[]  IntegratorOutMax=[]  FilterOutMin=[]  FilterOutMax=[]  SumI1OutMin=[]  SumI1OutMax=[]  SumI2OutMin=[]  SumI2OutMax=[]  SumI3OutMin=[]  SumI3OutMax=[]  SumI4OutMin=[]  SumI4OutMax=[]  SumDOutMin=[]  SumDOutMax=[]  DifferentiatorOutMin=[]  DifferentiatorOutMax=[]  FilterDiffOutCoefMin=[]  FilterDiffOutCoefMax=[]  ReciprocalOutMin=[]  ReciprocalOutMax=[]  SumDenOutMin=[]  SumDenOutMax=[]  SumNumOutMin=[]  SumNumOutMax=[]  DivideOutMin=[]  DivideOutMax=[]  UdiffTsProdOutMin=[]  UdiffTsProdOutMax=[]  NTsProdOutMin=[]  NTsProdOutMax=[]  UintegralTsProdOutMin=[]  UintegralTsProdOutMax=[]  UngainTsProdOutMin=[]  UngainTsProdOutMax=[]  ClampingZeroOutDataTypeStr=Inherit: Inherit via back propagation  ClampingZeroOutMin=[]  ClampingZeroOutMax=[]  FilterDenConstantOutDataTypeStr=Inherit: Inherit via back propagation  FilterDenConstantOutMin=[]  FilterDenConstantOutMax=[]  PCopyOutDataTypeStr=Inherit: Inherit via back propagation  PCopyOutMin=[]  PCopyOutMax=[]  NCopyOutDataTypeStr=Inherit: Inherit via back propagation  NCopyOutMin=[]  NCopyOutMax=[]  IntegratorContinuousStateAttributes=''  IntegratorStateMustResolveToSignalObject=off  IntegratorRTWStateStorageClass=Auto  FilterContinuousStateAttributes=''  FilterStateMustResolveToSignalObject=off  FilterRTWStateStorageClass=Auto  ParallelPVariant=InternalParameters  IdealPVariant=Disabled  IVariant=Disabled  DVariant=Disabled  IntegratorVariant=Disabled  SatVariant=Disabled  AWVariant=Disabled  PCopyVariant=Disabled  TRVariant=Disabled  FdbkBlocksVariant=Forward  IdealPFdbkVariant=Disabled  SatFdbkVariant=Disabled  DerivativeFilterVariant=Disabled  NVariant=Disabled  NCopyVariant=Disabled_SignalSpec  FilterICVariant=Disabled  IntegratorICVariant=Disabled  ExternalResetVariant=Disabled  TRSumVariant=Passthrough  SumFdbkVariant=Disabled  SumVariant=Passthrough_P  TsampFilterVariant=InternalTs  TsampNgainVariant=Passthrough  TsampIntegralVariant=Disabled_SignalSpec  ExternalSaturationOutDataTypeStr=Inherit: Same as second input
  Sum : Sum  Inputs=|+-
  throttle : Outport
  wires:
  Vb/1 -> "Incidence, Sideslip, & Airspeed"/1
  "Incidence, Sideslip, & Airspeed"/3 -> Sum/2
  Command_Speed/1 -> Sum/1
  Sum/1 -> PID Controller/1
  PID Controller/1 -> Add/2
  Constant/1 -> Add/1
  Constant1/1 -> Mux/3
  Constant2/1 -> Mux/4
  Add/1 -> Mux/2, Mux/1
  Mux/1 -> throttle/1

== system Project_Mobius/EVTOL Model/6DOF Dynamics/Attitude_Function ==
  pqr : Inport
  attitude : Inport  Port=2
  Add : Sum
  Add1 : Sum
  Cos : Trigonometry  Operator=cos
  Demux : Demux  Outputs=3
  Demux1 : Demux  Outputs=3
  Mux : Mux  Inputs=3
  Product{,1..6} (7 alike) : Product
  SinCos : Trigonometry  Operator=sincos
  Tan : Trigonometry  Operator=tan
  dot_phi : Sum
  dot_psi : Product  Inputs=/*
  dot_theta : Sum  Inputs=+-
  dot_attitude : Outport
  wires:
  pqr/1 -> Demux/1
  attitude/1 -> Demux1/1
  Demux1/2 -> Cos/1, Tan/1
  Demux1/1 -> SinCos/1
  Demux/3 -> Product5/1, Product4/1, Product/1
  SinCos/2 -> Product5/2, Product3/2, Product/2
  SinCos/1 -> Product4/2, Product6/2, Product1/2
  Demux/2 -> Product6/1, Product3/1, Product1/1
  Product/1 -> Add/2
  Product1/1 -> Add/1
  Tan/1 -> Product2/2
  Add/1 -> Product2/1
  Demux/1 -> dot_phi/1
  Product2/1 -> dot_phi/2
  Product3/1 -> dot_theta/1
  Product4/1 -> dot_theta/2
  Product5/1 -> Add1/1
  Product6/1 -> Add1/2
  Cos/1 -> dot_psi/1
  Add1/1 -> dot_psi/2
  dot_psi/1 -> Mux/3
  dot_theta/1 -> Mux/2
  dot_phi/1 -> Mux/1
  Mux/1 -> dot_attitude/1

== system Project_Mobius/EVTOL Model/6DOF Dynamics/Force_Function ==
  Vb : Inport
  F_Total : Inport  Port=2
  pqr : Inport  Port=3
  Demux : Demux  Outputs=3
  Demux1 : Demux  Outputs=3
  Demux2 : Demux  Outputs=3
  Gain : Gain  Gain=1/aircraft_mass
  Mux : Mux  Inputs=3
  Product{,1..5} (6 alike) : Product
  dot_u : Sum  Inputs=++-
  dot_v : Sum  Inputs=++-
  dot_w : Sum  Inputs=++-
  dot_Vb : Outport
  wires:
  Vb/1 -> Demux/1
  pqr/1 -> Demux1/1
  F_Total/1 -> Gain/1
  Demux/2 -> Product5/1, Product/1
  Demux1/3 -> Product2/2, Product/2
  Demux/3 -> Product3/1, Product1/1
  Demux1/2 -> Product4/2, Product1/2
  Gain/1 -> Demux2/1
  Product1/1 -> dot_u/3
  Product/1 -> dot_u/2
  Demux2/1 -> dot_u/1
  Demux/1 -> Product4/1, Product2/1
  Demux1/1 -> Product5/2, Product3/2
  Product3/1 -> dot_v/2
  Demux2/2 -> dot_v/1
  Product2/1 -> dot_v/3
  Product4/1 -> dot_w/2
  Product5/1 -> dot_w/3
  Demux2/3 -> dot_w/1
  dot_u/1 -> Mux/1
  dot_v/1 -> Mux/2
  dot_w/1 -> Mux/3
  Mux/1 -> dot_Vb/1

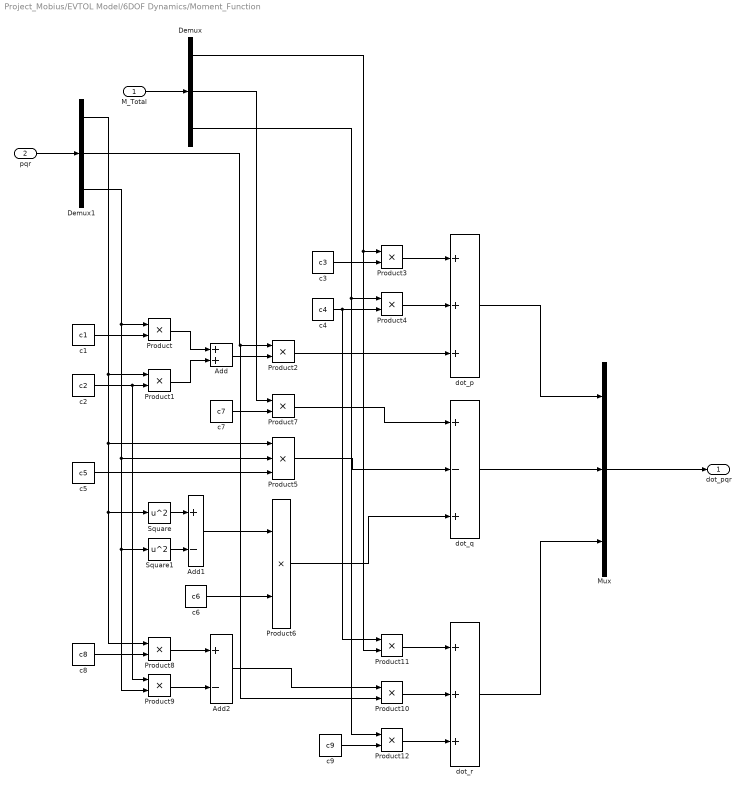
== system Project_Mobius/EVTOL Model/6DOF Dynamics/Moment_Function ==
  M_Total : Inport
  pqr : Inport  Port=2
  Add : Sum
  Add1 : Sum  Inputs=+-
  Add2 : Sum  Inputs=+-
  Demux : Demux  Outputs=3
  Demux1 : Demux  Outputs=3
  Mux : Mux  Inputs=3
  Product{,1..4,6..12} (12 alike) : Product
  Product5 : Product  Inputs=3
  Square : Math  Operator=square
  Square1 : Math  Operator=square
  c1 : Constant  Value=c1
  c2 : Constant  Value=c2
  c3 : Constant  Value=c3
  c4 : Constant  Value=c4
  c5 : Constant  Value=c5
  c6 : Constant  Value=c6
  c7 : Constant  Value=c7
  c8 : Constant  Value=c8
  c9 : Constant  Value=c9
  dot_p : Sum  Inputs=+++
  dot_q : Sum  Inputs=+-+
  dot_r : Sum  Inputs=+++
  dot_pqr : Outport
  wires:
  M_Total/1 -> Demux/1
  pqr/1 -> Demux1/1
  c1/1 -> Product/2
  Demux1/3 -> Product9/2, Square1/1, Product5/2, Product/1
  c2/1 -> Product9/1, Product1/2
  Demux1/1 -> Square/1, Product8/1, Product5/1, Product1/1
  Product1/1 -> Add/2
  Product/1 -> Add/1
  Add/1 -> Product2/2
  Demux1/2 -> Product10/2, Product2/1
  c3/1 -> Product3/2
  Demux/1 -> Product3/1, Product11/2
  Demux/3 -> Product4/1, Product12/1
  c4/1 -> Product11/1, Product4/2
  Product2/1 -> dot_p/3
  Product4/1 -> dot_p/2
  Product3/1 -> dot_p/1
  c5/1 -> Product5/3
  Square/1 -> Add1/1
  Square1/1 -> Add1/2
  Add1/1 -> Product6/1
  c6/1 -> Product6/2
  c7/1 -> Product7/2
  Demux/2 -> Product7/1
  Product7/1 -> dot_q/1
  Product5/1 -> dot_q/2
  Product6/1 -> dot_q/3
  c8/1 -> Product8/2
  Product8/1 -> Add2/1
  Product9/1 -> Add2/2
  Add2/1 -> Product10/1
  c9/1 -> Product12/2
  Product11/1 -> dot_r/1
  Product10/1 -> dot_r/2
  Product12/1 -> dot_r/3
  dot_q/1 -> Mux/2
  dot_r/1 -> Mux/3
  dot_p/1 -> Mux/1
  Mux/1 -> dot_pqr/1
